simulink model "turbulence_VonKarmanModel"  (R2014a)
settings: Solver=ode45  StartTime=0.0  StopTime=10  MaxStep=0.01  RelTol=1e-3
values from neighbouring files (symbols this model uses):
  turbolenceParameters = initTurbulenceParameters(h,turbolenceParameters,severityChoosed)    [comparingModels.m]
  Va = input('Choose aircraft airspeed [m/s]\nVa=')    [comparingModels.m]
libraries: simulink x1
settings Model: Creator=Domenico  LastModifiedBy=Domenico

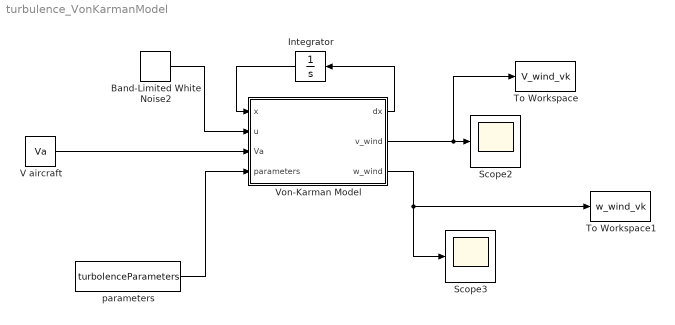
== system turbulence_VonKarmanModel ==
  Band-Limited White Noise2 : simulink/Sources/Band-Limited White Noise  Cov=[0.1]  Ts=0.1  seed=[23341]
  Integrator : Integrator  InitialCondition=zeros(17,1)'
  Scope2 : Scope
      settings: ShowLegends=on
  Scope3 : Scope
      settings: ShowLegends=on  SaveName=ScopeData3
  To Workspace : ToWorkspace  VariableName=V_wind_vk  SaveFormat=Structure With Time  SampleTime=-1
  To Workspace1 : ToWorkspace  VariableName=w_wind_vk  SaveFormat=Structure With Time  SampleTime=-1
  V aircraft : Constant  Value=Va
  Von-Karman Model : MATLAB Function  TreatAsAtomicUnit=on
  parameters : Constant  Value=turbolenceParameters  OutDataTypeStr=Bus: myParamsType
  wires:
  Integrator/1 -> Von-Karman Model/1(x)
  Von-Karman Model/1(dx) -> Integrator/1
  Band-Limited White Noise2/1 -> Von-Karman Model/2(u)
  V aircraft/1 -> Von-Karman Model/3(Va)
  Von-Karman Model/3(w_wind) -> Scope3/1, To Workspace1/1
  Von-Karman Model/2(v_wind) -> To Workspace/1, Scope2/1
  parameters/1 -> Von-Karman Model/4(parameters)

== matlab function turbulence_VonKarmanModel/Von-Karman Model ==
  data: x input; u input; dx output; Va input; parameters input; v_wind output; w_wind output
function [dx,v_wind,w_wind]  = fcn(x,u,Va,parameters)
%This function returns V_wind and w_wind vectors by linear and angular
%velocity of wind - Von-Karman Model

%   Form: fcn(x,u,parameters,V)
%   Inputs :    x              -> state
%               u              -> white noise
%               parameters     -> vector parameters
%               V              -> velocity aircraft
%   Outputs :   V_wind         -> linear speed wind [u,v,w]
%               w_wind         -> angular rate wind [p,q,r]
%               dx             -> differential state

%% State component
ux   = x(1); % longitudinal u-component (TRANSLATIONAL COMPONENT)
uxd  = x(2); % derived u-component
vx   = x(3); % lateral v-component (TRANSLATIONAL COMPONENT)
vxd  = x(4); % derived v-component
vx2d = x(5); % second derived of v-component
wx   = x(6); % vertical w-component(TRANSLATIONAL COMPONENT)
wxd  = x(7); % derived w-component
wx2d = x(8); % second derived of w-component
px   = x(9); % Longitudinal p-component (ROTATIONAL COMPONENT)
rx   = x(10); % Lateral r-component (ROTATIONAL COMPONENT)
rxd  = x(11); % derived of r-component
rx2d = x(12); % second derived of r-component
rx3d = x(13); % third derived of r-component
qx   = x(14);% vertical q-component (ROTATIONAL COMPONENT)
qxd  = x(15);% derived of p-component
qx2d = x(16);% second derived of p-component
qx3d = x(17);% third derived of p-component
%% Input 
eta = u; % white noise

%% Parameters
% %turbolence intensities
sigma_u = parameters.sigma_u;
sigma_v = parameters.sigma_v;
sigma_w = parameters.sigma_w;
% %scale lengths
Lu      = parameters.Lu;
Lv      = parameters.Lv;
Lw      = parameters.Lw;
b       = parameters.b; %wing span

%% Util terms
a1Term = sigma_u*sqrt(2/pi*Lu/Va);
b1Term = 0.25*Lu/Va;
c1Term = 1.357*Lu/Va;
d1Term = 0.1987 *(Lu/Va)^2;
a2Term = sigma_v*sqrt(1/pi*Lv/Va);
b2Term = 2.7478*Lv/Va;
c2Term = 0.3398*(Lv/Va)^2;
d2Term = 2.9958*Lv/Va;
e2Term = 1.9754*(Lv/Va)^2;
f2Term = 0.1539*(Lv/Va)^3;
a3Term = sigma_w*sqrt(1/pi*Lw/Va);
b3Term = 2.7478*Lw/Va;
c3Term = 0.3398*(Lw/Va)^2;
d3Term = 2.9958*Lw/Va;
e3Term = 1.9754*(Lw/Va)^2;
f3Term = 0.1539*(Lw/Va)^3;
a4Term = (sigma_w*sqrt(0.8/Va)*(pi/(4*b)^(1/6)))/(Lw^(1/3));
b4Term = (4*b)/(pi*Va);
a5Term = (3*b)/(pi*Va);

dx=[uxd;
   -(ux/d1Term) - ((c1Term*uxd)/d1Term)+ eta;
   vxd;
   vx2d;
   -(vx/f2Term) - ((d2Term*vxd)/f2Term) - ((e2Term*vx2d)/f2Term) + eta;
   wxd;
   wx2d;
   -(wx/f3Term) - ((d3Term*wxd)/f3Term) - ((e3Term*wx2d)/f3Term) + eta;
   -px/b4Term+eta;
   rxd;
   rx2d;
   rx3d;
   eta-(rx/(f2Term*a5Term))-((a2Term+a5Term)*rxd)/(f2Term*a5Term)-((e2Term+d2Term*a5Term)*rx2d)/(f2Term*a5Term)-((f2Term+e2Term*a5Term)*rx3d)/(f2Term*a5Term);
   qxd;
   qx2d;
   qx3d;
   eta-(qx/(f3Term*b4Term))-((a3Term+b4Term)*qxd)/(f3Term*b4Term)-((e3Term+d3Term*b4Term)*qx2d)/(f3Term*b4Term)-((f3Term+e3Term*b4Term)*qx3d)/(f3Term*b4Term)];
 

%% Translational component of wind 
ugw = (a1Term/d1Term)*ux+((a1Term*b1Term)/d1Term)*uxd;                                   % Longitudinal
vgw = (a2Term/f2Term)*vx+((a2Term*b2Term)/f2Term)*vxd+((a2Term*c2Term)/f2Term)*vx2d;     % Lateral
wgw = (a3Term/f3Term)*wx+((a3Term*b3Term)/f3Term)*wxd+((a3Term*c3Term)/f3Term)*wx2d;     % Vertical

%% Rotational component of wind 
pgw = (a4Term/b4Term)*px;                                                                                                 % Longitudinal
rgw = (a2Term/(f2Term*a5Term*Va))*rxd+((a2Term*b2Term)/(f2Term*a5Term*Va))*rx2d + ((a2Term*c2Term)/(f2Term*a5Term*Va))*rx3d;  % Lateral
qgw = (a3Term/(f3Term*b4Term*Va))*qxd+((a3Term*b3Term)/(f3Term*b4Term*Va))*qx2d + ((a3Term*c3Term)/(f3Term*b4Term*Va))*qx3d;   % Vertical

v_wind=[ugw;vgw;wgw];
w_wind=[pgw;qgw;rgw];
end
